simulink model "bh_6dof_quat_integrate"  (R2019b)
settings: Solver=ode45  StartTime=0.0  StopTime=200  FixedStep=0.001  EnableMultiTasking=on
undefined symbols (not defined in the file or in its folder): P_elec, P_mot, P_one_prop, P_rot, P_veh, sigbuilder_block
libraries: bh_6dof_LIBRARY x23, simulink_extras x20, simulink x16
(part 3 of 3)

== system bh_6dof_quat_integrate/CONT_SYS W_MOT_CMDS/MOTOR_sys/MOTOR_1/prefilter ==
  note: Y = U *     wn^2/( s^2 + 2*p*wn*s + wn^2)
      | Y*( s^2 + 2*p*wn*s + wn^2) = U * wn^2
      |
      | y'' + y'*2*p*wn + y*wn^2 = U*wn^2
  U : Inport
  Gain : Gain  Gain=2*p*wn
  Gain1 : Gain  Gain=wn^2
  Gain2 : Gain  Gain=wn^2
  Integrator : Integrator
  Integrator1 : Integrator
  Sum : Sum  Inputs=|+--
  U_filt : Outport
  U_DOT : Outport  Port=2
  wires:
  Integrator/1 -> Integrator1/1, [Y_DOT], Gain/1  "y_dot"
  Sum/1 -> Integrator/1  "y_dot_dot"
  Integrator1/1 -> Gain1/1, U_filt/1  "y"
  U/1 -> Gain2/1
  Gain2/1 -> Sum/1
  Gain/1 -> Sum/3
  Gain1/1 -> Sum/2
  [Y_DOT] -> U_DOT/1

== system bh_6dof_quat_integrate/CONT_SYS W_MOT_CMDS/MOTOR_sys/MOTOR_2/prefilter ==
  note: Y = U *     wn^2/( s^2 + 2*p*wn*s + wn^2)
      | Y*( s^2 + 2*p*wn*s + wn^2) = U * wn^2
      |
      | y'' + y'*2*p*wn + y*wn^2 = U*wn^2
  U : Inport
  Gain : Gain  Gain=2*p*wn
  Gain1 : Gain  Gain=wn^2
  Gain2 : Gain  Gain=wn^2
  Integrator : Integrator
  Integrator1 : Integrator
  Sum : Sum  Inputs=|+--
  U_filt : Outport
  U_DOT : Outport  Port=2
  wires:
  Integrator/1 -> Integrator1/1, [Y_DOT], Gain/1  "y_dot"
  Sum/1 -> Integrator/1  "y_dot_dot"
  Integrator1/1 -> Gain1/1, U_filt/1  "y"
  U/1 -> Gain2/1
  Gain2/1 -> Sum/1
  Gain/1 -> Sum/3
  Gain1/1 -> Sum/2
  [Y_DOT] -> U_DOT/1

== system bh_6dof_quat_integrate/CONT_SYS W_MOT_CMDS/MOTOR_sys/MOTOR_3/prefilter ==
  note: Y = U *     wn^2/( s^2 + 2*p*wn*s + wn^2)
      | Y*( s^2 + 2*p*wn*s + wn^2) = U * wn^2
      |
      | y'' + y'*2*p*wn + y*wn^2 = U*wn^2
  U : Inport
  Gain : Gain  Gain=2*p*wn
  Gain1 : Gain  Gain=wn^2
  Gain2 : Gain  Gain=wn^2
  Integrator : Integrator
  Integrator1 : Integrator
  Sum : Sum  Inputs=|+--
  U_filt : Outport
  U_DOT : Outport  Port=2
  wires:
  Integrator/1 -> Integrator1/1, [Y_DOT], Gain/1  "y_dot"
  Sum/1 -> Integrator/1  "y_dot_dot"
  Integrator1/1 -> Gain1/1, U_filt/1  "y"
  U/1 -> Gain2/1
  Gain2/1 -> Sum/1
  Gain/1 -> Sum/3
  Gain1/1 -> Sum/2
  [Y_DOT] -> U_DOT/1

== system bh_6dof_quat_integrate/CONT_SYS W_MOT_CMDS/MOTOR_sys/MOTOR_4/prefilter ==
  note: Y = U *     wn^2/( s^2 + 2*p*wn*s + wn^2)
      | Y*( s^2 + 2*p*wn*s + wn^2) = U * wn^2
      |
      | y'' + y'*2*p*wn + y*wn^2 = U*wn^2
  U : Inport
  Gain : Gain  Gain=2*p*wn
  Gain1 : Gain  Gain=wn^2
  Gain2 : Gain  Gain=wn^2
  Integrator : Integrator
  Integrator1 : Integrator
  Sum : Sum  Inputs=|+--
  U_filt : Outport
  U_DOT : Outport  Port=2
  wires:
  Integrator/1 -> Integrator1/1, [Y_DOT], Gain/1  "y_dot"
  Sum/1 -> Integrator/1  "y_dot_dot"
  Integrator1/1 -> Gain1/1, U_filt/1  "y"
  U/1 -> Gain2/1
  Gain2/1 -> Sum/1
  Gain/1 -> Sum/3
  Gain1/1 -> Sum/2
  [Y_DOT] -> U_DOT/1

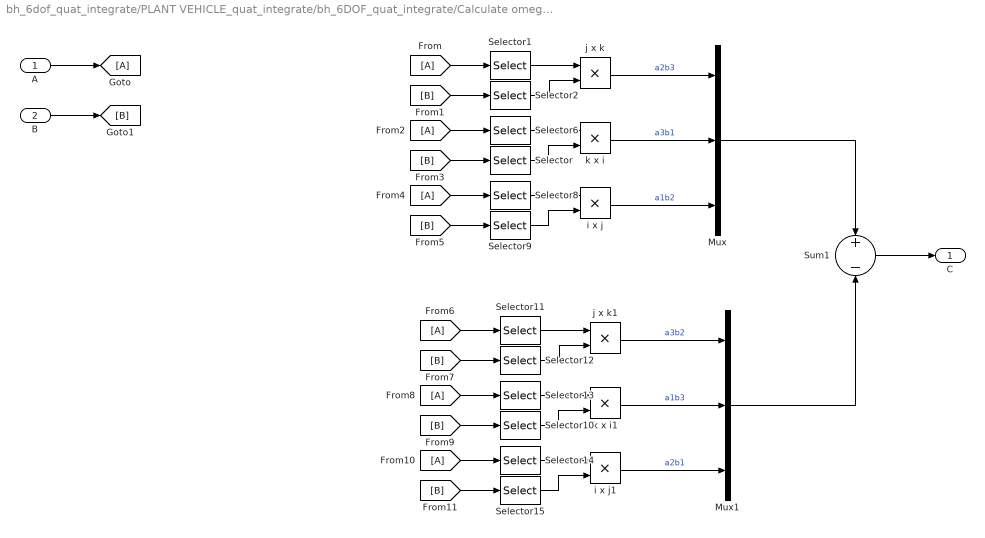
== system bh_6dof_quat_integrate/PLANT VEHICLE_quat_integrate/bh_6DOF_quat_integrate/Calculate omega_dot/w_x_(I.w) ==
  A : Inport
  B : Inport  Port=2
  Mux : Mux  Inputs=3
  Mux1 : Mux  Inputs=3
  Selector{,8,13,15} (4 alike) : Selector  InputPortWidth=3  IndexOptions=Index vector (dialog)  Indices=1  OutputSizes=1
  Selector{1,9,12,14} (4 alike) : Selector  InputPortWidth=3  IndexOptions=Index vector (dialog)  Indices=2  OutputSizes=1
  Selector{2,6,10..11} (4 alike) : Selector  InputPortWidth=3  IndexOptions=Index vector (dialog)  Indices=3  OutputSizes=1
  Sum1 : Sum  Inputs=+|-  SaturateOnIntegerOverflow=on  InputSameDT=on  OutDataTypeStr=Inherit: Same as first input
  i x j : Product  SaturateOnIntegerOverflow=on  InputSameDT=on  OutDataTypeStr=Inherit: Same as first input
  i x j1 : Product  SaturateOnIntegerOverflow=on  InputSameDT=on  OutDataTypeStr=Inherit: Same as first input
  j x k : Product  SaturateOnIntegerOverflow=on  InputSameDT=on  OutDataTypeStr=Inherit: Same as first input
  j x k1 : Product  SaturateOnIntegerOverflow=on  InputSameDT=on  OutDataTypeStr=Inherit: Same as first input
  k x i : Product  SaturateOnIntegerOverflow=on  InputSameDT=on  OutDataTypeStr=Inherit: Same as first input
  k x i1 : Product  SaturateOnIntegerOverflow=on  InputSameDT=on  OutDataTypeStr=Inherit: Same as first input
  C : Outport
  wires:
  Selector15/1 -> i x j1/2
  Selector14/1 -> i x j1/1
  [B] -> Selector15/1
  [A] -> Selector14/1
  Selector10/1 -> k x i1/2
  Selector13/1 -> k x i1/1
  [B] -> Selector10/1
  [A] -> Selector13/1
  [A] -> Selector11/1
  [B] -> Selector12/1
  Selector12/1 -> j x k1/2
  Selector11/1 -> j x k1/1
  Mux1/1 -> Sum1/2
  j x k1/1 -> Mux1/1  "a3b2"
  k x i1/1 -> Mux1/2  "a1b3"
  i x j1/1 -> Mux1/3  "a2b1"
  Selector9/1 -> i x j/2
  Selector8/1 -> i x j/1
  [B] -> Selector9/1
  [A] -> Selector8/1
  Selector/1 -> k x i/2
  Selector6/1 -> k x i/1
  [B] -> Selector/1
  [A] -> Selector6/1
  [A] -> Selector1/1
  [B] -> Selector2/1
  A/1 -> [A]
  B/1 -> [B]
  Selector2/1 -> j x k/2
  Selector1/1 -> j x k/1
  Sum1/1 -> C/1
  Mux/1 -> Sum1/1
  j x k/1 -> Mux/1  "a2b3"
  k x i/1 -> Mux/2  "a3b1"
  i x j/1 -> Mux/3  "a1b2"

== system bh_6dof_quat_integrate/PLANT VEHICLE_quat_integrate/bh_6DOF_quat_integrate/Integrate_QUAT/Calc Euler_rates ==
  "p q r " : Inport
  Euler_angs : Inport  Port=2
  Demux1 : Demux  Outputs=3
  Demux2 : Demux  Outputs=3
  Demux3 : Demux  Outputs=3
  Mux1 : Mux  Inputs=3
  Reshape1 : Reshape  OutputDimensionality=Column vector (2-D)
  Reshape2 : Reshape  OutputDimensionality=Column vector (2-D)
  Terminator : Terminator
  my_euler_rates : MATLAB Function  TreatAsAtomicUnit=on
  Euler_rates : Outport
  wires:
  Demux1/3 -> my_euler_rates/2(psi)  "psi"
  Demux1/1 -> Terminator/1  "phi"
  Demux1/2 -> my_euler_rates/1(theta)  "theta"
  "p q r "/1 -> Reshape1/1
  Euler_angs/1 -> Demux1/1
  Demux3/1 -> my_euler_rates/3(p)
  Demux3/2 -> my_euler_rates/4(q)
  Demux3/3 -> my_euler_rates/5(r)
  Mux1/1 -> Reshape2/1
  Reshape2/1 -> Euler_rates/1
  Demux2/1 -> Mux1/1  "phidot_Z1_yaw"
  Demux2/2 -> Mux1/2  "thetadot_Y2_pitch"
  Demux2/3 -> Mux1/3  "psidot_X3_roll"
  my_euler_rates/1(euler_rates) -> Demux2/1  "euler_rates"
  Reshape1/1 -> Demux3/1  "wb"

== system bh_6dof_quat_integrate/PLANT VEHICLE_quat_integrate/bh_6DOF_quat_integrate/Integrate_QUAT/NORMLIZE_occasionally ==
  note: One strategy for NORMALIZING the quaternion
  note: eg: every 10 seconds normalize
  In1 : Inport
  Adjust_to_UNITY : Subsystem
  Out1 : Outport
  wires:
  In1/1 -> Adjust_to_UNITY/1(qin)
  Adjust_to_UNITY/1(q_unit) -> Out1/1

== system bh_6dof_quat_integrate/PLANT VEHICLE_quat_integrate/bh_6DOF_quat_integrate/Integrate_QUAT/NORMLIZE_occasionally/Adjust_to_UNITY ==
  note: Every 10 seconds normalize
      | the quaternion to ensure it is a
      | UNIT quaternion
  qin : Inport
  Data Type Conversion : DataTypeConversion  OutDataTypeStr=double
  Detect Increase : simulink/Logic and Bit Operations/Detect Increase  vinit=0.0  OutDataTypeStr=boolean
  MATLAB Function : MATLAB Function  TreatAsAtomicUnit=on
  Pulse Generator : DiscretePulseGenerator  PulseType=Time based  Period=10  PulseWidth=50
  Scope : Scope
  q_unit : Outport
  wires:
  Pulse Generator/1 -> Detect Increase/1
  Detect Increase/1 -> Data Type Conversion/1
  MATLAB Function/1(q) -> q_unit/1
  Data Type Conversion/1 -> MATLAB Function/1(change_signal)
  qin/1 -> MATLAB Function/2(q_in)
  MATLAB Function/2(mag_of_q) -> Scope/1

== matlab function bh_6dof_quat_integrate/PLANT VEHICLE_quat_integrate/bh_6DOF_quat_integrate/Integrate_QUAT/Calc Euler_rates/my_euler_rates ==
  data: theta input; euler_rates output; psi input; p input; q input; r input
function euler_rates = my_euler_rates(theta,psi,p,q,r)
%#codegen

%    This function was generated by the Symbolic Math Toolbox version 7.0.
%    09-Jun-2016 10:28:25

euler_rates = [(r.*cos(psi)+q.*sin(psi))./cos(theta);
                q.*cos(psi)-r.*sin(psi);
               (p.*cos(theta)+r.*cos(psi).*sin(theta)+q.*sin(psi).*sin(theta))./cos(theta)];

== matlab function bh_6dof_quat_integrate/CONT_SYS W_MOT_CMDS/FM_to_w2 ==
  data: L input; w2_cmd output; Thrust_const input; Twist_const input; Thrust input; TQ_roll_X input; TQ_pit_Y input; TQ_yaw_Z input
function w2_cmd = FMtow2(L, Thrust_const, Twist_const, Thrust, TQ_roll_X, TQ_pit_Y, TQ_yaw_Z)
%#codegen

    % simplify the variable names
    b = Thrust_const;
    k = Twist_const;

    % construct the co-efficient matrix:
    %  F_and_M = C * w^2
    %
    % C = [     b,    b,    b,    b;
    %           0,    b*L,  0,   -b*L;
    %          -b*L,  0,    b*L,  0;
    %          -k,    k,   -k,    k; ];

    % used Symbolic toolbox to compute inv(C)
    C_inv = [
             1/(4*b),          0, -1/(2*L*b), -1/(4*k);
             1/(4*b),  1/(2*L*b),          0,  1/(4*k);
             1/(4*b),          0,  1/(2*L*b), -1/(4*k);
             1/(4*b), -1/(2*L*b),          0,  1/(4*k);
            ];
    % solve for the w^2 vec
    F_and_M_col = [Thrust, TQ_roll_X, TQ_pit_Y, TQ_yaw_Z].' ;

    w2_cmd = C_inv * F_and_M_col;
    
    tf_col = (w2_cmd >= 0);
   assert(all(w2_cmd), 'ERROR: some w2 are NEGATIVE !')
   %assert(false, 'ERROR: some w2 are NEGATIVE !')
end

== matlab function bh_6dof_quat_integrate/CONT_SYS W_MOT_CMDS/w2toFM ==
  data: L input; Thrust output; Thrust_const input; Twist_const input; w2_col input; TQ_roll_X output; TQ_pit_Y output; TQ_yaw_Z output
function [Thrust, TQ_roll_X, TQ_pit_Y, TQ_yaw_Z] = w2toFM(L, Thrust_const, Twist_const, w2_col)
%#codegen

    % simplify the variable names
    b = Thrust_const;
    k = Twist_const;

    % construct the co-efficient matrix:
    %  F_and_M = C * w^2
    
    C = [     b,    b,    b,    b;
              0,    b*L,  0,   -b*L;
             -b*L,  0,    b*L,  0;
             -k,    k,   -k,    k; ];

    % solve for the FM_col
    %   FM_col = [Thrust, TQ_roll_X, TQ_pit_Y, TQ_yaw_Z].' ;
    
    FM_col  =  C * w2_col;
    
    Thrust    =  FM_col(1);
    TQ_roll_X =  FM_col(2);
    TQ_pit_Y  =  FM_col(3);
    TQ_yaw_Z  =  FM_col(4);
    
end

== matlab function bh_6dof_quat_integrate/CONT_SYS Force_Moment_CMDS/PITCH_and_ROLL_CONT/MATLAB Function ==
  data: Gr input size=[2 1]; Qr output size=[2 1]; ang input size=[1 1]
function Qr = fcn(Gr, ang)
%#codegen

    bRg = [  cos(ang),  sin(ang);
            -sin(ang),  cos(ang);
          ];  

    Qr = bRg * Gr;
end

== matlab function bh_6dof_quat_integrate/PLANT VEHICLE_quat_integrate/bh_6DOF_quat_integrate/Integrate_QUAT/NORMLIZE_occasionally/Adjust_to_UNITY/MATLAB Function ==
  data: change_signal input double size=1; q output; q_in input double size=[4 1]; mag_of_q output
function [q, mag_of_q] = fcn(change_signal, q_in)

if(change_signal > 0.5)
    q = q_in / norm(q_in);
else
    q = q_in;
end

mag_of_q = norm(q);

end

== matlab function bh_6dof_quat_integrate/PLANT VEHICLE_quat_integrate/bh_6DOF_quat_integrate/Integrate_QUAT/calc_bRg ==
  data: q_col input double size=[4, 1]; bRg output double size=[3 3]
function bRg = fcn(q_col)

% VERY SLOW in SIMULINK
%--------------------------------------------------------------
%   coder.extrinsic('bh_api_for_SL_model_calc_bRg') 
%
%   bRg = bh_api_for_SL_model_calc_bRg(q_col);
%--------------------------------------------------------------

    q0    = q_col(1);
    qx    = q_col(2);
    qy    = q_col(3);
    qz    = q_col(4);
    
    % *** PROOF: bh_explore_eigenaxis_AND_quat_DCM_derivation.mlx ***
    %            (it is s trivial substitution from this result)
    C_11  = qx^2 + q0^2 - qy^2 - qz^2;
    C_12  = 2*(qx*qy + qz*q0);
    C_13  = 2*(qx*qz - qy*q0);
       
    C_21  = 2*(qx*qy - qz*q0);
    C_22  = qy^2 + q0^2 - qx^2 - qz^2;
    C_23  = 2*(qy*qz + qx*q0);
    
    C_31  = 2*(qx*qz + qy*q0);
    C_32  = 2*(qy*qz - qx*q0);
    C_33  = qz^2 + q0^2 - qx^2 - qy^2;
    
    
    bRg = [ C_11, C_12, C_13;
            C_21, C_22, C_23;
            C_31, C_32, C_33;   ];   


end

== matlab function bh_6dof_quat_integrate/PLANT VEHICLE_quat_integrate/bh_6DOF_quat_integrate/Integrate_QUAT/MATLAB Function2 ==
  data: bRg input; phi output; theta output; psi output
function [phi, theta, psi] = calc_EUL_angs(bRg)
%#codegen

%NOTE:  this is bRg ... and NOT gRb

% bRg = [ ...
%                               cos(phi)*cos(theta),                              cos(theta)*sin(phi),         -sin(theta);
%  cos(phi)*sin(psi)*sin(theta) - cos(psi)*sin(phi), cos(phi)*cos(psi) + sin(phi)*sin(psi)*sin(theta), cos(theta)*sin(psi);
%  sin(phi)*sin(psi) + cos(phi)*cos(psi)*sin(theta), cos(psi)*sin(phi)*sin(theta) - cos(phi)*sin(psi), cos(psi)*cos(theta);
%  ];

theta = asin( -bRg(1,3) );
phi   = atan2(   bRg(1,2)/cos(theta), bRg(1,1)/cos(theta) ); % <--- SINGULARITY @ theta=pi/2
psi   = atan2(   bRg(2,3)/cos(theta), bRg(3,3)/cos(theta) ); % <--- SINGULARITY @ theta=pi/2
end

== matlab function bh_6dof_quat_integrate/PLANT VEHICLE_quat_integrate/bh_6DOF_quat_integrate/Integrate_QUAT/calc_q_DOT ==
  data: q_col input double size=[4, 1]; q_dot_col output double size=[4 1]; wb_col input double size=[3, 1]
function q_dot_col = fcn(q_col, wb_col)

% VERY SLOW in SIMULINK
%--------------------------------------------------------------
% coder.extrinsic('bh_api_for_SL_model_calc_QDOT')
%
% q_dot_col = bh_api_for_SL_model_calc_QDOT(q_col, wb_col);
%--------------------------------------------------------------

% *** PROOF: bh_explore_eigenaxis_AND_quat_rates.mlx ***    
q0     = q_col(1);
qx     = q_col(2);
qy     = q_col(3);
qz     = q_col(4);

A      = [  -qx,  -qy,  -qz;
             q0,  -qz,   qy;
             qz,   q0,  -qx;
            -qy,   qx,   q0;  ];

wb_col = wb_col(:);

q_dot_col  = 0.5 * A * wb_col;


end
